simulink library "LopesDevelopmentLibrary"  (R2015b)
settings: Solver=ode45  StartTime=0.0  StopTime=10.0  RelTol=1e-3
values from neighbouring files (symbols this model uses):
  d2r = @(d) d*(pi/180)    [LopesDevelopmentLibrary_LoadParameters.m]
  ts = LopesParams.ts    [LopesDevelopmentLibrary_LoadParameters.m]
undefined symbols (not defined in the file or in its folder): anyParameterChanged, DiscIntNeverNeededParam, gcbh, LAP, LHF, LKF, LopesParams, macaddr, mxpcnetworkconfig, mxpcrtudprx, mxpcrtudptx, patientParametersChanged, port, PX, PZ, RAP, RHF, RKF, SelectorLOPESInSize, StrideTime_s, Time
undefined symbols (not defined in the file): LopesParamsSendDataArrayLen
libraries: LopesDevelopmentLibrary x327, simulink x100, dspmtrx3 x49, xpciplib x6, xpcnetworkbufferlib x5, dspsigops x4, dspstat3 x3, xpcethernetlib x2, visionstatistics x2, xpcseriallib x2, LopesDevelopmentLibraryTest x1, nmc x1
(part 1 of 12)
settings Model: xpc_rtwmakecfg_data=_xpcnblib__xpciplib__xpcetherlib__xpcether8255xlib__xpcetherGbElib_  Creator=Administrator  LastModifiedBy=brugtjh
settings DataIOCC: SaveFormat=Array  SignalLoggingSaveFormat=ModelDataLogs
settings OptimizationCC: ExpressionDepthLimit=2147483647
settings DebuggingCC: UnderspecifiedInitializationDetection=Classic  MergeDetectMultiDrivingBlocksExec=none  SolverPrmCheckMsg=warning  FcnCallInpInsideContextMsg=UseLocalSettings  StateNameClashWarn=warning
settings HardwareCC: ProdBitPerPointer=32  ProdLargestAtomicFloat=None  ProdIntDivRoundTo=Undefined  ProdEndianess=Unspecified  ProdWordSize=32  ProdHWDeviceType=32-bit Generic
settings GRTTargetCC: GeneratePreprocessorConditionals=Disable all  CombineOutputUpdateFcns=off  GRTInterface=on
settings ConfigComp: CovModelRefEnable=Off

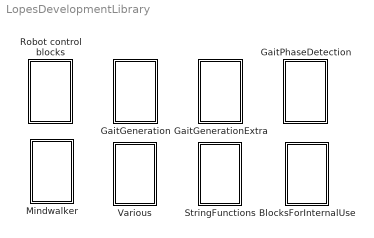
== system LopesDevelopmentLibrary ==
  BlocksForInternalUse : Subsystem
  GaitGeneration : Subsystem
  GaitGenerationExtra : Subsystem
  GaitPhaseDetection : Subsystem
  Mindwalker : Subsystem
  Robot control blocks : Subsystem
  StringFunctions : Subsystem
  Various : Subsystem

== system LopesDevelopmentLibrary/BlocksForInternalUse ==
  GaitGeneration : Subsystem
  GaitGenerationStartStop : Subsystem
  LLC Communication : Subsystem

== system LopesDevelopmentLibrary/GaitGeneration ==
  CalculateBreaksCoefs : Subsystem  TreatAsAtomicUnit=on
  CalculateReferenceStiffnesses : Subsystem
  ConvertStiffness : Subsystem
  GaitParameters : Subsystem
  GeneratePhaseSignalNoFeedback : Subsystem
  GenerateReferenceTrajectory : Subsystem
  PatientParameters : Subsystem
  PhaseEstimatorAoyagi : Subsystem  mask{Weights=[1.0, 0.3, 1.0, 0.3, 0.1, 0, 0.1, 0], AoyagiFilterGain=5}
      mask prompts: Weights "Weights (LHF LKF RHF RKF dLHF dLKF dRHF dRKF) (default: [1.0, 0.3, 1.0, 0.3, 0.1, 0, 0.1, 0])"; AoyagiFilterGain "Aoyagi Filter Gain (default: 5)"
  PhaseEstimatorAoyagi_wPI : Subsystem  mask{Weights=[1.0, 0.1, 1.0, 0.1, 0.0, 0, 0.0, 0], AoyagiFilterGain=2, AoyagiIntegralTimeConstant=5}
      mask prompts: Weights "Weights (LHF LKF RHF RKF dLHF dLKF dRHF dRKF) (default: [1.0, 0.3, 1.0, 0.3, 0.1, 0, 0.1, 0])"; AoyagiFilterGain "Aoyagi Filter Gain (default: 5)"; AoyagiIntegralTimeConstant "Aoyagi Integral Time Constant"

== system LopesDevelopmentLibrary/GaitGenerationExtra ==
  CalculateBreaksCoefs : Subsystem  TreatAsAtomicUnit=on
  GaitGenerationAndAnalysis : Subsystem
      settings: MinAlgLoopOccurrences=on
  GaitParameters : Subsystem
  PhaseEstimatorAoyagi_wPI_Extra : Subsystem  mask{Weights=[1.0, 0.1, 1.0, 0.1, 0.0, 0, 0.0, 0], AoyagiFilterGain=2, AoyagiIntegralTimeConstant=5}
      mask prompts: Weights "Weights (LHF LKF RHF RKF dLHF dLKF dRHF dRKF) (default: [1.0, 0.3, 1.0, 0.3, 0.1, 0, 0.1, 0])"; AoyagiFilterGain "Aoyagi Filter Gain (default: 5)"; AoyagiIntegralTimeConstant "Aoyagi Integral Time Constant"
  VelocityHold : Subsystem

== system LopesDevelopmentLibrary/GaitPhaseDetection ==
  Gait Phase Detection with Wrapper : Subsystem
  Gait Phase detection : Subsystem

== system LopesDevelopmentLibrary/Mindwalker ==
  Mindwalker_AdaptiveTreadmillVelocity : Subsystem
  Mindwalker_Lopes_Conversion : Subsystem

== system LopesDevelopmentLibrary/Robot control blocks ==
  FromLopes : Subsystem
  GeneralLopes : Subsystem  LoadFcn=LopesDevelopmentLibrary_LoadParameters
  RS232SyncBox : Subsystem
  ToLopes : Subsystem

== system LopesDevelopmentLibrary/StringFunctions ==
  Pad : Subsystem  mask{outArrayLen=100}
      mask prompts: outArrayLen "Size of output array"
  PadStrAsDouble : Subsystem  mask{outArrayLen=LopesParams.exceptionStrArrayLen}
      mask prompts: outArrayLen "Size of output array"
  ShowStringInMatlabConsoleIfNotEmpty : MATLAB Function  TreatAsAtomicUnit=on
  concat : MATLAB Function  TreatAsAtomicUnit=on
  concat3 : MATLAB Function  TreatAsAtomicUnit=on
  concat5 : Subsystem  mask{outStrLen=LopesParamsSendDataArrayLen}
      mask prompts: outStrLen "Length of output array"
  concatDelimiter : MATLAB Function  TreatAsAtomicUnit=on
  concatWithOptionalDelimiter : MATLAB Function  TreatAsAtomicUnit=on
  strlen : MATLAB Function  TreatAsAtomicUnit=on
  strlen_as_double : MATLAB Function  TreatAsAtomicUnit=on

== system LopesDevelopmentLibrary/Various ==
  note: Note: I have had problems
      | with real boolean constants
      | in xPC Target. Consider
      | using the Boolean1, which ouptuts
      | a double (and can be converted to boolean
      | if you need to).
  AddToMatrixColumn : Subsystem  mask{col=1, minimum=-inf, maximum=inf}
      mask prompts: col "Column (1-based)"
      mask Display:
      | plot([15,10,10,15],[0,0,75,75])
      | plot([70,75,75,70],[0,0,75,75])
      | plot(0,-5)
      | plot(85,85)
      | plot([55,55],[60,70])
      | plot([50,60],[65,65])
      | plot([55,55],[35,45])
      | plot([50,60],[40,40])
      | plot([55,55],[10,20])
      | plot([50,60],[15,15])
  AddToMatrixElement : Subsystem  mask{row=1, col=1, minimum=-inf, maximum=inf}
      mask prompts: row "Row (1-based)"; col "Column (1-based)"
      mask Display:
      | plot([15,10,10,15],[0,0,75,75])
      | plot([70,75,75,70],[0,0,75,75])
      | plot(0,-5)
      | plot(85,85)
      | plot([55,55],[70,60])
      | plot([50,60],[65,65])
  AdjustAmplitude : Subsystem
  AnyChanged : Subsystem
  AssignMatrixElement : Subsystem  mask{row=3, col=2, minimum=-inf, maximum=inf}
      mask prompts: row "Row (1-based)"; col "Column (1-based)"; minimum "Minimum value"; maximum "Maximum value"
      mask Display:
      | plot([15,10,10,15],[0,0,75,75])
      | plot([70,75,75,70],[0,0,75,75])
      | plot(0,-5)
      | plot(85,85)
      | plot([50,60,60,50,50],[60,60,70,70,60])
  BetterSpringVelocities : Subsystem
  Boolean : Constant  Value=false  OutDataTypeStr=boolean
      settings: OpenFcn=|
      | b = get_param(gcb,'value');
      | if (strcmp(b,'true')),
      |   set_param (gcb,'value','false');
      | else
      |   set_param(gcb,'value','true');
      | end;
  Boolean1 : Constant  Value=0  OutDataTypeStr=double
      settings: OpenFcn=|
      | b = get_param(gcb,'value');
      | if (strcmp(b,'1')),
      |   set_param (gcb,'value','0');
      | else
      |   set_param(gcb,'value','1');
      | end;
  CompareAny : Subsystem  mask{values=[3,4]}
      mask Display: disp(['==(',num2strjoin(values,'||'),')'])
  CrossFade : Subsystem
  CrossfadeInNSeconds : Subsystem
  Cycloid : Subsystem
  Decimation : Subsystem  mask{Decimation=1}
      mask prompts: Decimation "Decimation Amount"
      mask TypeOptions Decimation: DecimationAmount/Value
      mask Display: disp(['Decimation: ',num2str(eval(get_param([gcb,'/DecimationAmount'],'Value')))])
  FilteredDerivative : Subsystem  mask{w=10*(2*pi), z=0.7}
      mask prompts: w "Cut off omega [rad/s]"; z "Zeta"
  FirstOrderLowPassFilter : Subsystem  mask{Tau=1}
  GenerateSyncPulseFromPhase : Subsystem
  IsFirstSample : Subsystem  InitFcn=|
      | return; %Disable this becasue it doesnt work!                                                                                                                                                          
      | h = gcb;                                                                                                                                                                                               
      | n = 0; % Number of enable blocks detected upstream                                                                                                                                                     
      | t = []; % type of enable blocks                                                                                                                                                                        
      | while 1,                                                                                                                                                                                               
      |   % Find parent                                                                                                                                                                                        
      |   h = get_param(h,'parent');                                                                                                                                                                           
      |   if (strcmp(h,'')),                                                                                                                                                                                   
      |       % Then we've reached the root                                                                                                                                                                    
      |       break;                                                                                                                                                                                           
      |   end;                                                                                                                                                                                                 
      |   % and check if it has an enable port                                                                                                                                                                 
      |   e = find_system(h,'searchdepth',1, 'BlockType','EnablePort');                                                                                                                                        
      |   if (numel(e)==1),                                                                                                                                                                                    
      |     s = get_param(e{1},'StatesWhenEnabling');                                                                                                                                                          
      |     n=n+1;                                                                                                                                                                                             
      |     if (strcmp(s,'held')),                                                                                                                                                                             
      |         t=[t;'h']; %#ok<AGROW>                                                                                                                                                                         
      |     else                                                                                                                                                                                               
      |         t=[t;'r']; %#ok<AGROW>                                                                                                                                                                         
      |     end;                                                                                                                                                                                               
      |   elseif (numel(e)>1),                                                                                                                                                                                 
      |       error('hun? Multiple enable blocks!')                                                                                                                                                            
      |   end;                                                                                                                                                                                                 
      | end;                                                                                                                                                                                                   
      |                                                                                                                                                                                                        
      | if (n==0),                                                                                                                                                                                             
      |     warning('Warning: %s - The block is not inside an enabled block',gcb)                                                                                                                              
      | elseif (n==1),                                                                                                                                                                                         
      |     if (t(1)=='r')                                                                                                                                                                                     
      |         % This is okay, do nothing                                                                                                                                                                     
      |     else                                                                                                                                                                                               
      |         warning('Warning: %s - This block is inside an enabled block which has its "State when enabling" set to "held". Usually you want it set to "reset" for correct operation.',gcb);               
      |     end;                                                                                                                                                                                               
      | else % n>1                                                                                                                                                                                             
      |     warning('Warning: %s - This block is inside multiple nested enabled blocks. Check which blocks are "held" and which are "reset". You usually want to have at least one "reset" enabled block',gcb);
      | end;
  Latch : Subsystem  mask{ic=0}
      mask prompts: ic "Initial Condition"
  MonoStable : Constant  Value=0
      settings: OpenFcn=set_param(gcb,'Value','1');tname = ['toggletimer_' gcb];delete(timerfind('name',tname));t = timer('timerfcn', ['set_param(''',gcb,''',''Value'',''0'')'],'executionmode','singleshot','startdelay',3,'name',tname);start(t);
      mask Display: fprintf('PushToTrigger\n%s',get_param(gcb,'value'))
  MultiplyMatrixElement : Subsystem  mask{row=1, col=1, minimum=-inf, maximum=inf}
      mask prompts: row "Row (1-based)"; col "Column (1-based)"; minimum "Minimum value"; maximum "Maximum value"
      mask Display:
      | plot([15,10,10,15],[0,0,75,75])
      | plot([70,75,75,70],[0,0,75,75])
      | plot(0,-5)
      | plot(85,85)
      | plot([50,60],[70,60])
      | plot([50,60],[60,70])
  PhaseShifter1 : Subsystem
  PhaseShifter2 : Subsystem
  PhaseWrapper : Subsystem
  PhaseWrapperAroundZero : Subsystem
  RateLimiterWithBypass : Subsystem  mask{up=3, down=-3}
      mask prompts: up "Rising slew rate:"; down "Falling slew rate:"
      mask help: If Bypass is nonzero, the rate-limiting functionality is bypassed, and the output is made equal to the input immediately.
  RateLimiterWithReset : Subsystem
  RelayCardControl : S-Function  FunctionName=PCI_1761_Relay  Parameters=baseaddress  SFunctionDeploymentMode=off  EnableBusSupport=off  mask{baseaddress=hex2dec('e000')}
      mask prompts: baseaddress "PCI Base Address (e.g. 0x0300)"
  SLRTMessage : Subsystem
  SafeDivide : Subsystem
      mask Display:
      | port_label('input',1,'X')
      | port_label('input',2,'/')
      | port_label('output',1,'')
  Sample Number Generator : Subsystem
      mask Display: disp('Sample Number\nGenerator')
  SampleNoStore : DataStoreMemory  DataStoreName=SAMPLENO  ReadBeforeWriteMsg=warning  WriteAfterWriteMsg=warning  WriteAfterReadMsg=warning
  SampleNumber : Subsystem
  SecondOrderHighPassFilter : Subsystem  mask{w=10*(2*pi), z=0.7}
      mask prompts: w "Cut off omega [rad/s]"; z "Zeta"
  SecondOrderLowPassFilter : Subsystem  mask{w=10*(2*pi), z=0.7}
      mask prompts: w "Cut off omega [rad/s]"; z "Zeta"
  Split : Subsystem
  Stopwatch : Subsystem
  TriggerAtPhaseCrossing : Subsystem
  WeightedAverage : Subsystem

== system LopesDevelopmentLibrary/BlocksForInternalUse/GaitGeneration ==
  CalculateCartesianPositions : Subsystem
  CalculateReferenceGait : Subsystem  TreatAsAtomicUnit=on
  CalculateStiffnessForOneJoint : Subsystem
  OrderKeyEvents : Subsystem
  RegressionData2KeyEvents : Subsystem
  SmoothlyRemove2ndKE : Subsystem
  TrajectoryOfInfluence : Subsystem
  keyEvents2breakscoefs3 : Subsystem  TreatAsAtomicUnit=on
      mask Display:
      | port_label('input',1,'keyEvents')
      | port_label('output',1,'breaks')
      | port_label('output',2,'coefs')
      | disp('keyEvents2breaksCoefs\n3rd order')
  keyEvents2breakscoefs5 : Subsystem  TreatAsAtomicUnit=on
      mask Display:
      | port_label('input',1,'keyEvents')
      | port_label('output',1,'breaks')
      | port_label('output',2,'coefs')
      | disp('keyEvents2breaksCoefs\n5th order')
  ppval_bus : Subsystem  TreatAsAtomicUnit=on

== system LopesDevelopmentLibrary/BlocksForInternalUse/GaitGenerationStartStop ==
  AddUselessKE : Subsystem
  AddUselessKEValue : Subsystem
  CalculateKEforStartup : Subsystem
  "ExtraKeyPoints " : Subsystem  mask{ExtraData='StartLeft', ConnectionPoint=100, SetVelocity=0.3, SetStrideTime=2}
      mask prompts: ExtraData "Name of the extra parameters (IE StartupLeft)"; ConnectionPoint "Connection point:"; SetVelocity "Set Velocity: (0 =  use current velocity)"; SetStrideTime "Set Stride Time: (0 =  use current stride time)"
      mask init:
      | set_param([gcb,'/PelvisTPX/RegressionData'],'Value',['LopesParams.GaitData',ExtraData,'.PX'])
      | set_param([gcb,'/PelvisTPZ/RegressionData'],'Value',['LopesParams.GaitData',ExtraData,'.PZ'])
      | 
      | set_param([gcb,'/LeftHipFlexion/RegressionData'],'Value',['LopesParams.GaitData',ExtraData,'.LHF'])
      | set_param([gcb,'/LeftKneeFlexion/RegressionData'],'Value',['LopesParams.GaitData',ExtraData,'.LKF'])
      | set_param([gcb,'/LeftAnklePF/RegressionData'],'Value',['LopesParams.GaitData',ExtraData,'.LAP'])
      | 
      | set_param([gcb,'/RightHipFlexion/RegressionData'],'Value',['LopesParams.GaitData',ExtraData,'.RHF'])
      | set_param([gcb,'/RightKneeFlexion/RegressionData'],'Value',['LopesParams.GaitData',ExtraData,'.RKF'])
      | set_param([gcb,'/RightAnklePF/RegressionData'],'Value',['LopesParams.GaitData',ExtraData,'.RAP'])
      mask DialogControl DescTextVar Prompt: This Mask sets the Settings for the extra added KeyPoints
  OrderKeyEventsAddOne : Subsystem

== system LopesDevelopmentLibrary/BlocksForInternalUse/LLC Communication ==
  LLC Network Configuration : Subsystem
  LLCReceiveUDP : Subsystem  mask{port=LopesParams.Communication.channel1ReceivePort}
      mask prompts: port "Receive port"
  LLCSendUDP : Subsystem  mask{port=LopesParams.Communication.channel1SendPort}
      mask prompts: port "Send port"
  UDP_Blocks : Subsystem
      mask Display: disp('')

== system LopesDevelopmentLibrary/GaitGeneration/CalculateBreaksCoefs ==
  Parameters : Inport
  Bus Assignment : BusAssignment  AssignedSignals=AnyValueHasChanged
  Bus Selector : BusSelector  OutputSignals=anyParameterChanged
  Calculate : Subsystem
  Data Type Conversion : DataTypeConversion  OutDataTypeStr=double
  BreaksCoefs : Outport  InitialOutput=0
  KeyEventTimes : Outport  Port=2
  Error : Outport  Port=3
  wires:
  Data Type Conversion/1 -> Bus Assignment/2
  Parameters/1 -> Bus Selector/1, Calculate/1(Parameters)
  Calculate/1(BreaksCoefs) -> Bus Assignment/1
  Calculate/2(KeyEventTimes) -> KeyEventTimes/1
  Calculate/3(Error) -> Error/1
  Bus Selector/1 -> Calculate/Enable, Data Type Conversion/1  "<anyParameterChanged>"
  Bus Assignment/1 -> BreaksCoefs/1

== system LopesDevelopmentLibrary/GaitGeneration/CalculateReferenceStiffnesses ==
  note: LHA1 and RHA1 can be used as a starting point
      | for stiffness implementation. They don't work as desired for now,
      | because stiffness for foot placement should increased
      | before heel contact; the key event from LAnkleZ which is used
      | inside the block, is too late.
  Phase : Inport
  KeyEventTimes : Inport  Port=2
  Parameters : Inport  Port=3
  Bus Selector{1,3..15} (14 alike) : BusSelector  OutputSignals=GuidanceForce_pct
  Bus Selector : BusSelector  OutputSignals=RAP,RKF,RHF,LAP,LKF,LHF
  Bus Selector2 : BusSelector  OutputSignals=General,WeightShift,LeftStepHeight,LeftCircumduction,LeftStabilityStance,LeftPrepositioning,LeftSteplength,LeftPushoff,RightStepHeight,RightCircumduction,RightStabilityStance,RightPrepositioning,RightSteplength,RightPushoff
  LAP : Subsystem
  LHA : Subsystem
  LHA1 : Subsystem  Commented=on
  LHF : Subsystem
  LKF : Subsystem
  Mux : Mux  Inputs=10
  PX : Subsystem
  PZ : Subsystem
  RAP : Subsystem
  RHA : Subsystem
  RHA1 : Subsystem  Commented=on
  RHF : Subsystem
  RKF : Subsystem
  Terminator : Terminator
  Terminator1 : Terminator
  Stiffness_pct : Outport
  wires:
  KeyEventTimes/1 -> Bus Selector/1
  Bus Selector15/1 -> Terminator1/1  "<GuidanceForce_pct>"
  Bus Selector14/1 -> Terminator/1  "<GuidanceForce_pct>"
  Bus Selector2/10 -> Bus Selector15/1  "<RightCircumduction>"
  Bus Selector2/4 -> Bus Selector14/1  "<LeftCircumduction>"
  Parameters/1 -> Bus Selector2/1
  Bus Selector4/1 -> PZ/2(WeightShift_GuidanceForce), LHA/1(WeightShift_GuidanceForce), RHA/1(WeightShift_GuidanceForce)  "<GuidanceForce_pct>"
  Bus Selector3/1 -> PZ/1(General_GuidanceForce), LHF/1(General_GuidanceForce), LKF/1(General_GuidanceForce), LAP/1(General_GuidanceForce), RHF/1(General_GuidanceForce), RKF/1(General_GuidanceForce), RAP/1(General_GuidanceForce), PX/1(General_GuidanceForce)  "<GuidanceForce_pct>"
  Mux/1 -> Stiffness_pct/1
  Phase/1 -> RHF/3(phase), RAP/3(phase), RKF/3(phase), LAP/3(phase), LHF/3(phase), LKF/3(phase)
  Bus Selector/5 -> LKF/2(breaks)  "<LKF>"
  Bus Selector/6 -> LHF/2(breaks)  "<LHF>"
  Bus Selector/3 -> RHF/2(breaks)  "<RHF>"
  Bus Selector/2 -> RKF/2(breaks)  "<RKF>"
  LKF/1(Stiffness_pct) -> Mux/5
  LHF/1(Stiffness_pct) -> Mux/4
  RHA/1(Stiffness_pct) -> Mux/7
  LHA/1(Stiffness_pct) -> Mux/3
  RHF/1(Stiffness_pct) -> Mux/8
  PZ/1(Stiffness_pct) -> Mux/2
  RKF/1(Stiffness_pct) -> Mux/9
  PX/1(Stiffness_pct) -> Mux/1
  Bus Selector2/1 -> Bus Selector3/1  "<General>"
  Bus Selector2/2 -> Bus Selector4/1  "<WeightShift>"
  Bus Selector2/3 -> Bus Selector1/1  "<LeftStepHeight>"
  Bus Selector2/6 -> Bus Selector5/1  "<LeftPrepositioning>"
  Bus Selector2/7 -> Bus Selector7/1  "<LeftSteplength>"
  Bus Selector2/9 -> Bus Selector8/1  "<RightStepHeight>"
  Bus Selector2/12 -> Bus Selector9/1  "<RightPrepositioning>"
  Bus Selector2/13 -> Bus Selector11/1  "<RightSteplength>"
  Bus Selector5/1 -> LAP/5(FootPlacement_GuidanceForce), LKF/6(FootPlacement_GuidanceForce), LHF/4(FootPlacement_GuidanceForce)  "<GuidanceForce_pct>"
  Bus Selector7/1 -> LHF/5(StepLength_GuidanceForce)  "<GuidanceForce_pct>"
  Bus Selector1/1 -> LAP/4(StepHeight_GuidanceForce), LKF/4(StepHeight_GuidanceForce)  "<GuidanceForce_pct>"
  Bus Selector13/1 -> LKF/5(StabilityInStance_GuidanceForce)  "<GuidanceForce_pct>"
  Bus Selector2/5 -> Bus Selector13/1  "<LeftStabilityStance>"
  Bus Selector2/11 -> Bus Selector12/1  "<RightStabilityStance>"
  Bus Selector9/1 -> RHF/4(FootPlacement_GuidanceForce), RKF/6(FootPlacement_GuidanceForce), RAP/5(FootPlacement_GuidanceForce)  "<GuidanceForce_pct>"
  Bus Selector11/1 -> RHF/5(StepLength_GuidanceForce)  "<GuidanceForce_pct>"
  Bus Selector8/1 -> RKF/4(StepHeight_GuidanceForce), RAP/4(StepHeight_GuidanceForce)  "<GuidanceForce_pct>"
  Bus Selector12/1 -> RKF/5(StabilityInStance_GuidanceForce)  "<GuidanceForce_pct>"
  RAP/1(Stiffness_pct) -> Mux/10
  LAP/1(Stiffness_pct) -> Mux/6
  Bus Selector/4 -> LAP/2(breaks)  "<LAP>"
  Bus Selector/1 -> RAP/2(breaks)  "<RAP>"
  Bus Selector2/8 -> Bus Selector6/1  "<LeftPushoff>"
  Bus Selector6/1 -> LAP/6(PushOff_GuidanceForce)  "<GuidanceForce_pct>"
  Bus Selector2/14 -> Bus Selector10/1  "<RightPushoff>"
  Bus Selector10/1 -> RAP/6(PushOff_GuidanceForce)  "<GuidanceForce_pct>"

== system LopesDevelopmentLibrary/GaitGeneration/ConvertStiffness ==
  note: This block converts from stiffness-in-percent to stiffness in Nm/rad and N/m.
      | The conversion from Stiffness_pct to Stiffness is nonlinear:
      | S = (S_pct/100)^gamma * MaxStiffness.
  Stiffness_pct : Inport
  ApplyGamma : Math  Operator=pow  SaturateOnIntegerOverflow=on
  Gamma : Constant  Value=LopesParams.Stiffness.Gamma
  MaximumJointStiffness : Constant  Value=LopesParams.Stiffness.MaxJointStiffness
  Product : Product  RndMeth=Zero
  ToFraction : Gain  Gain=0.01
  Stiffness : Outport  LockScale=on
  wires:
  Product/1 -> Stiffness/1
  ApplyGamma/1 -> Product/2
  ToFraction/1 -> ApplyGamma/1
  MaximumJointStiffness/1 -> Product/1
  Gamma/1 -> ApplyGamma/2
  Stiffness_pct/1 -> ToFraction/1

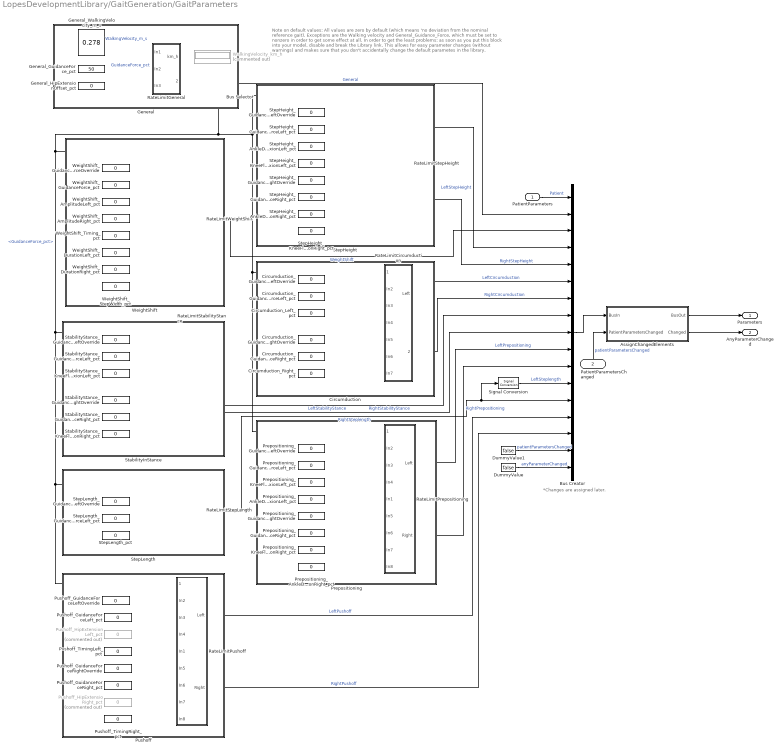
== system LopesDevelopmentLibrary/GaitGeneration/GaitParameters ==
  note: Note on default values:
      | All values are zero by default (which means 'no deviation from the nominal reference gait).
      | Exceptions are the Walking velocity and General_Guidance_Force, which must be
      | set to nonzero in order to get some effect at all.
      |
      | In order to get the least problems: as soon as you put this block into your model, disable and
      | break the Library link. This allows for easy parameter changes (without warnings) and makes
      | sure that you don't accidentally change the default parametes in the library.
  note: *Changes are assigned later.
  PatientParameters : Inport
  PatientParametersChanged : Inport  Port=2
  AssignChangedElements : Subsystem
  Bus Creator : BusCreator  Inputs=17
  Bus Selector : BusSelector  OutputSignals=GuidanceForce_pct
  Circumduction : Subsystem
  Circumduction_GuidanceForceLeftOverride : Constant  Value=0  OutDataTypeStr=double
      settings: OpenFcn=|
      | b = get_param(gcb,'value');
      | if (strcmp(b,'1')),
      |   set_param (gcb,'value','0');
      | else
      |   set_param(gcb,'value','1');
      | end;
  Circumduction_GuidanceForceLeft_pct : Constant  Value=0
  Circumduction_GuidanceForceRightOverride : Constant  Value=0  OutDataTypeStr=double
      settings: OpenFcn=|
      | b = get_param(gcb,'value');
      | if (strcmp(b,'1')),
      |   set_param (gcb,'value','0');
      | else
      |   set_param(gcb,'value','1');
      | end;
  Circumduction_GuidanceForceRight_pct : Constant  Value=0
  Circumduction_Left_pct : Constant  Value=0
  Circumduction_Right_pct : Constant  Value=0
  DummyValue : Constant  Value=false  OutDataTypeStr=boolean
  DummyValue1 : Constant  Value=false
  General : Subsystem
  General_GuidanceForce_pct : Constant  Value=50
  General_HipExtensionOffset_pct : Constant  Value=0
  General_WalkingVelocity_m_s : Constant  Value=0.278
  Prepositioning : Subsystem
  Prepositioning_AnkleDorsiFlexionLeft_pct : Constant  Value=0
  Prepositioning_AnkleDorsiFlexionRight_pct : Constant  Value=0
  Prepositioning_GuidanceForceLeftOverride : Constant  Value=0  OutDataTypeStr=double
      settings: OpenFcn=|
      | b = get_param(gcb,'value');
      | if (strcmp(b,'1')),
      |   set_param (gcb,'value','0');
      | else
      |   set_param(gcb,'value','1');
      | end;
  Prepositioning_GuidanceForceLeft_pct : Constant  Value=0
  Prepositioning_GuidanceForceRightOverride : Constant  Value=0  OutDataTypeStr=double
      settings: OpenFcn=|
      | b = get_param(gcb,'value');
      | if (strcmp(b,'1')),
      |   set_param (gcb,'value','0');
      | else
      |   set_param(gcb,'value','1');
      | end;
  Prepositioning_GuidanceForceRight_pct : Constant  Value=0
  Prepositioning_KneeFlexionLeft_pct : Constant  Value=0
  Prepositioning_KneeFlexionRight_pct : Constant  Value=0
  Pushoff : Subsystem
  Pushoff_GuidanceForceLeftOverride : Constant  Value=0  OutDataTypeStr=double
      settings: OpenFcn=|
      | b = get_param(gcb,'value');
      | if (strcmp(b,'1')),
      |   set_param (gcb,'value','0');
      | else
      |   set_param(gcb,'value','1');
      | end;
  Pushoff_GuidanceForceLeft_pct : Constant  Value=0
  Pushoff_GuidanceForceRightOverride : Constant  Value=0  OutDataTypeStr=double
      settings: OpenFcn=|
      | b = get_param(gcb,'value');
      | if (strcmp(b,'1')),
      |   set_param (gcb,'value','0');
      | else
      |   set_param(gcb,'value','1');
      | end;
  Pushoff_GuidanceForceRight_pct : Constant  Value=0
  Pushoff_HipExtensioRight_pct : Constant  Commented=on  Value=0
  Pushoff_HipExtensionLeft_pct : Constant  Commented=on  Value=0
  Pushoff_TimingLeft_pct : Constant  Value=0
  Pushoff_TimingRight_pct : Constant  Value=0
  RateLimitCircumduction : Subsystem
  RateLimitGeneral : Subsystem
  RateLimitPrepositioning : Subsystem
  RateLimitPushoff : Subsystem
  RateLimitStabilityStance : Subsystem
  RateLimitStepHeight : Subsystem
  RateLimitStepLength : Subsystem
  RateLimitWeightShift : Subsystem
  Signal Conversion : SignalConversion
  StabilityInStance : Subsystem
  StabilityStance_GuidanceForceLeftOverride : Constant  Value=0  OutDataTypeStr=double
      settings: OpenFcn=|
      | b = get_param(gcb,'value');
      | if (strcmp(b,'1')),
      |   set_param (gcb,'value','0');
      | else
      |   set_param(gcb,'value','1');
      | end;
  StabilityStance_GuidanceForceLeft_pct : Constant  Value=0
  StabilityStance_GuidanceForceRightOverride : Constant  Value=0  OutDataTypeStr=double
      settings: OpenFcn=|
      | b = get_param(gcb,'value');
      | if (strcmp(b,'1')),
      |   set_param (gcb,'value','0');
      | else
      |   set_param(gcb,'value','1');
      | end;
  StabilityStance_GuidanceForceRight_pct : Constant  Value=0
  StabilityStance_KneeFlexionLeft_pct : Constant  Value=0
  StabilityStance_KneeFlexionRight_pct : Constant  Value=0
  StepHeight : Subsystem
  StepHeight_AnkleDorsiflexionLeft_pct : Constant  Value=0
  StepHeight_AnkleDorsiflexionRight_pct : Constant  Value=0
  StepHeight_GuidanceForceLeftOverride : Constant  Value=0  OutDataTypeStr=double
      settings: OpenFcn=|
      | b = get_param(gcb,'value');
      | if (strcmp(b,'1')),
      |   set_param (gcb,'value','0');
      | else
      |   set_param(gcb,'value','1');
      | end;
  StepHeight_GuidanceForceLeft_pct : Constant  Value=0
  StepHeight_GuidanceForceRightOverride : Constant  Value=0  OutDataTypeStr=double
      settings: OpenFcn=|
      | b = get_param(gcb,'value');
      | if (strcmp(b,'1')),
      |   set_param (gcb,'value','0');
      | else
      |   set_param(gcb,'value','1');
      | end;
  StepHeight_GuidanceForceRight_pct : Constant  Value=0
  StepHeight_KneeFlexionLeft_pct : Constant  Value=0
  StepHeight_KneeFlexionRight_pct : Constant  Value=0
  StepLength : Subsystem
  StepLength_GuidanceForceLeftOverride : Constant  Value=0  OutDataTypeStr=double
      settings: OpenFcn=|
      | b = get_param(gcb,'value');
      | if (strcmp(b,'1')),
      |   set_param (gcb,'value','0');
      | else
      |   set_param(gcb,'value','1');
      | end;
  StepLength_GuidanceForceLeft_pct : Constant  Value=0
  StepLength_pct : Constant  Value=0
  WalkingVelocity_km_h : Display  Commented=on
  WeightShift : Subsystem
  WeightShift_AmplitudeLeft_pct : Constant  Value=0
  WeightShift_AmplitudeRight_pct : Constant  Value=0
  WeightShift_DurationLeft_pct : Constant  Value=0
  WeightShift_DurationRight_pct : Constant  Value=0
  WeightShift_GuidanceForceOverride : Constant  Value=0  OutDataTypeStr=double
      settings: OpenFcn=|
      | b = get_param(gcb,'value');
      | if (strcmp(b,'1')),
      |   set_param (gcb,'value','0');
      | else
      |   set_param(gcb,'value','1');
      | end;
  WeightShift_GuidanceForce_pct : Constant  Value=0
  WeightShift_StepWidth_pct : Constant  Value=0
  WeightShift_Timing_pct : Constant  Value=0
  Parameters : Outport
  AnyParameterChanged : Outport  Port=2
  wires:
  AssignChangedElements/1(BusOut) -> Parameters/1
  Signal Conversion/1 -> Bus Creator/12  "LeftSteplength"
  DummyValue1/1 -> Bus Creator/16  "patientParametersChanged"
  DummyValue/1 -> Bus Creator/17  "anyParameterChanged"
  RateLimitWeightShift/1(Out1) -> Bus Creator/3  "WeightShift"
  PatientParameters/1 -> Bus Creator/1  "Patient"
  RateLimitStepHeight/1(Left) -> Bus Creator/4  "LeftStepHeight"
  RateLimitStepHeight/2(Right) -> Bus Creator/5  "RightStepHeight"
  RateLimitStabilityStance/1(Left) -> Bus Creator/8  "LeftStabilityStance"
  RateLimitStabilityStance/2(Right) -> Bus Creator/9  "RightStabilityStance"
  RateLimitPrepositioning/1(Left) -> Bus Creator/10  "LeftPrepositioning"
  RateLimitPrepositioning/2(Right) -> Bus Creator/11  "RightPrepositioning"
  RateLimitStepLength/1(StepLength) -> Bus Creator/13, Signal Conversion/1  "RightSteplength"
  RateLimitCircumduction/1(Left) -> Bus Creator/6  "LeftCircumduction"
  RateLimitCircumduction/2(Right) -> Bus Creator/7  "RightCircumduction"
  WeightShift_GuidanceForceOverride/1 -> RateLimitWeightShift/2(In2)
  WeightShift_GuidanceForce_pct/1 -> RateLimitWeightShift/3(In3)
  WeightShift_AmplitudeLeft_pct/1 -> RateLimitWeightShift/4(In4)
  WeightShift_AmplitudeRight_pct/1 -> RateLimitWeightShift/5(In5)
  WeightShift_Timing_pct/1 -> RateLimitWeightShift/6(In6)
  WeightShift_DurationLeft_pct/1 -> RateLimitWeightShift/7(In7)
  WeightShift_DurationRight_pct/1 -> RateLimitWeightShift/8(In8)
  WeightShift_StepWidth_pct/1 -> RateLimitWeightShift/9(In9)
  StepHeight_GuidanceForceLeftOverride/1 -> RateLimitStepHeight/2(In2)
  StepHeight_GuidanceForceLeft_pct/1 -> RateLimitStepHeight/3(In3)
  StepHeight_KneeFlexionLeft_pct/1 -> RateLimitStepHeight/5(In4)
  StepHeight_GuidanceForceRightOverride/1 -> RateLimitStepHeight/6(In5)
  StepHeight_GuidanceForceRight_pct/1 -> RateLimitStepHeight/7(In6)
  StepHeight_KneeFlexionRight_pct/1 -> RateLimitStepHeight/9(In7)
  Circumduction_GuidanceForceLeftOverride/1 -> RateLimitCircumduction/2(In2)
  Circumduction_GuidanceForceLeft_pct/1 -> RateLimitCircumduction/3(In3)
  Circumduction_Left_pct/1 -> RateLimitCircumduction/4(In4)
  Circumduction_GuidanceForceRightOverride/1 -> RateLimitCircumduction/5(In5)
  Circumduction_GuidanceForceRight_pct/1 -> RateLimitCircumduction/6(In6)
  Circumduction_Right_pct/1 -> RateLimitCircumduction/7(In7)
  StabilityStance_GuidanceForceLeftOverride/1 -> RateLimitStabilityStance/2(In2)
  StabilityStance_GuidanceForceLeft_pct/1 -> RateLimitStabilityStance/3(In3)
  StabilityStance_KneeFlexionLeft_pct/1 -> RateLimitStabilityStance/4(In4)
  StabilityStance_GuidanceForceRightOverride/1 -> RateLimitStabilityStance/5(In5)
  StabilityStance_GuidanceForceRight_pct/1 -> RateLimitStabilityStance/6(In6)
  StabilityStance_KneeFlexionRight_pct/1 -> RateLimitStabilityStance/7(In7)
  Prepositioning_GuidanceForceLeftOverride/1 -> RateLimitPrepositioning/2(In2)
  Prepositioning_GuidanceForceLeft_pct/1 -> RateLimitPrepositioning/3(In3)
  Prepositioning_KneeFlexionLeft_pct/1 -> RateLimitPrepositioning/4(In4)
  Prepositioning_GuidanceForceRightOverride/1 -> RateLimitPrepositioning/6(In5)
  Prepositioning_GuidanceForceRight_pct/1 -> RateLimitPrepositioning/7(In6)
  Prepositioning_KneeFlexionRight_pct/1 -> RateLimitPrepositioning/8(In7)
  StepLength_GuidanceForceLeftOverride/1 -> RateLimitStepLength/2(In2)
  StepLength_GuidanceForceLeft_pct/1 -> RateLimitStepLength/3(In3)
  StepLength_pct/1 -> RateLimitStepLength/4(In4)
  Bus Selector/1 -> RateLimitStepHeight/1(GeneralGF), RateLimitPrepositioning/1(GeneralGF), RateLimitCircumduction/1(GeneralGF), RateLimitWeightShift/1(GeneralGF), RateLimitPushoff/1(GeneralGF), RateLimitStepLength/1(GeneralGF), RateLimitStabilityStance/1(GeneralGF)  "<GuidanceForce_pct>"
  RateLimitGeneral/2(General) -> Bus Creator/2, Bus Selector/1  "General"
  General_WalkingVelocity_m_s/1 -> RateLimitGeneral/1(In1)  "WalkingVelocity_m_s"
  General_GuidanceForce_pct/1 -> RateLimitGeneral/2(In2)  "GuidanceForce_pct"
  General_HipExtensionOffset_pct/1 -> RateLimitGeneral/3(In3)
  RateLimitGeneral/1(km_h) -> WalkingVelocity_km_h/1
  Bus Creator/1 -> AssignChangedElements/1(BusIn)
  PatientParametersChanged/1 -> AssignChangedElements/2(PatientParametersChanged)  "patientParametersChanged"
  AssignChangedElements/2(Changed) -> AnyParameterChanged/1
  StepHeight_AnkleDorsiflexionLeft_pct/1 -> RateLimitStepHeight/4(In1)
  StepHeight_AnkleDorsiflexionRight_pct/1 -> RateLimitStepHeight/8(In8)
  Prepositioning_AnkleDorsiFlexionLeft_pct/1 -> RateLimitPrepositioning/5(In1)
  Prepositioning_AnkleDorsiFlexionRight_pct/1 -> RateLimitPrepositioning/9(In8)
  Pushoff_GuidanceForceLeft_pct/1 -> RateLimitPushoff/3(In3)
  Pushoff_HipExtensionLeft_pct/1 -> RateLimitPushoff/4(In4)
  Pushoff_GuidanceForceRightOverride/1 -> RateLimitPushoff/6(In5)
  Pushoff_GuidanceForceRight_pct/1 -> RateLimitPushoff/7(In6)
  Pushoff_HipExtensioRight_pct/1 -> RateLimitPushoff/8(In7)
  Pushoff_TimingLeft_pct/1 -> RateLimitPushoff/5(In1)
  Pushoff_TimingRight_pct/1 -> RateLimitPushoff/9(In8)
  RateLimitPushoff/1(Left) -> Bus Creator/14  "LeftPushoff"
  RateLimitPushoff/2(Right) -> Bus Creator/15  "RightPushoff"
  Pushoff_GuidanceForceLeftOverride/1 -> RateLimitPushoff/2(In2)

== system LopesDevelopmentLibrary/GaitGeneration/GeneratePhaseSignalNoFeedback ==
  note: This block is a very simple implementation
      | of a phase-signal generator. You can use this for testing.
      | However, don't use it for real experiments.
      |
      | It seems logical to fix the step time. However, the step length
      | and walking velocity are also fixed. The step time can be uniquely
      | determined from this. If we would also fix the step time, we'd get
      | an overdetermined system. In order to avoid, we need to
      | leave the step time free to change. Therefore, this block
      | (which fixes step time because it fixes phase evolution), should
      | not be used in reality.
  BreaksCoefs : Inport
  Bus Selector2 : BusSelector  OutputSignals=StrideTime_s
  Constant3 : Constant  Value=100
  Integrator : Integrator
  PhaseWrapper : LopesDevelopmentLibrary/Various/PhaseWrapper
  SafeDivide : LopesDevelopmentLibrary/Various/SafeDivide  SystemSampleTime=-1
  Phase_pct : Outport
  PhaseRate_pct_s : Outport  Port=2
  wires:
  BreaksCoefs/1 -> Bus Selector2/1
  Constant3/1 -> SafeDivide/1
  SafeDivide/1 -> Integrator/1, PhaseRate_pct_s/1
  Bus Selector2/1 -> SafeDivide/2  "<StrideTime_s>"
  Integrator/1 -> PhaseWrapper/1
  PhaseWrapper/1 -> Phase_pct/1

== system LopesDevelopmentLibrary/GaitGeneration/GenerateReferenceTrajectory ==
  Phase : Inport
  BreaksCoefs : Inport  Port=2
  Parameters : Inport  Port=3
  Bus Selector : BusSelector  OutputSignals=General.WalkingVelocity_m_s
  CalculateReferenceGait : LopesDevelopmentLibrary/BlocksForInternalUse/GaitGeneration/CalculateReferenceGait
  CopySignal : SignalConversion
  Terminator1 : Terminator
  Terminator2 : Terminator
  JointAngles : Outport
  JointAngularVelocities : Outport  Port=2
  JointAngularAccelerations : Outport  Port=3
  TreadmillVelocity : Outport  Port=4
  TimeSinceLeftHeelstrike : Outport  Port=5
  wires:
  CalculateReferenceGait/6 -> Terminator2/1
  CalculateReferenceGait/5 -> Terminator1/1
  CalculateReferenceGait/1 -> JointAngles/1
  Parameters/1 -> CalculateReferenceGait/3, Bus Selector/1
  BreaksCoefs/1 -> CalculateReferenceGait/2
  CopySignal/1 -> TreadmillVelocity/1
  Phase/1 -> CalculateReferenceGait/1
  CalculateReferenceGait/2 -> JointAngularVelocities/1
  CalculateReferenceGait/3 -> JointAngularAccelerations/1
  CalculateReferenceGait/4 -> TimeSinceLeftHeelstrike/1
  Bus Selector/1 -> CopySignal/1  "<WalkingVelocity_m_s>"

== system LopesDevelopmentLibrary/GaitGeneration/PatientParameters ==
  note: Warning: Only change these values while in state Off.
      | Otherwise, the result may be unexpected (things don't go
      | really wrong, but the results may be less accurate).
  note: Distance between hip joints
  note: Don't change (the ankle of Lopes is 0.1 m above the
      | ground, regardless of where the human's ankle is).
  note: this should be a little shorter than the
      | real foot length. 0.2 to 0.25 is usually best.
  AnyChanged : LopesDevelopmentLibrary/Various/AnyChanged
  BodyLength_m : Constant  Value=1.80
  Bus Creator : BusCreator  Inputs=8
  FootHeight_m : Constant  Value=0.10
  FootLength_m : Constant  Value=0.2
  LowerLegLength_m : Constant  Value=0.5
  Mass_kg : Constant  Value=80
  PelvisHeight_m : Constant  Value=0.2
  PelvisWidth_m : Constant  Value=0.2
  UpperLegLength_m : Constant  Value=0.5
  PatientParameters : Outport
  PatientParametersChanged : Outport  Port=2
  wires:
  PelvisHeight_m/1 -> Bus Creator/8  "PelvisHeight_m"
  PelvisWidth_m/1 -> Bus Creator/7  "PelvisWidth_m"
  FootHeight_m/1 -> Bus Creator/6  "FootHeight_m"
  BodyLength_m/1 -> Bus Creator/1  "BodyLength_m"
  Mass_kg/1 -> Bus Creator/5  "Mass_kg"
  Bus Creator/1 -> AnyChanged/1, PatientParameters/1
  UpperLegLength_m/1 -> Bus Creator/2  "UpperLegLength_m"
  LowerLegLength_m/1 -> Bus Creator/3  "LowerLegLength_m"
  FootLength_m/1 -> Bus Creator/4  "FootLength_m"
  AnyChanged/1 -> PatientParametersChanged/1

== system LopesDevelopmentLibrary/GaitGeneration/PhaseEstimatorAoyagi ==
  note: This block is a phase estimator based on the paper by Aoyagi 2007. It consists of two parts:
      | -  a raw estimator which estimates the current phase simply based on the euclidean distance
      |    to each point on the trajectory (it returns the phase at which this distance is minimum), and
      | - a (sort-of-low-pass)-filter which generates a continuous and not-too-fast-changing output phase.
  MeasuredJointAngles : Inport
  MeasuredJointVelocities : Inport  Port=2
  BreaksCoefs : Inport  Port=3
  ResetHighActive : Inport  Port=4
  Bus Selector : BusSelector  OutputSignals=StrideTime_s
  EstimatePhaseDirectlyAoyagi : Subsystem
  PhaseFilterAoyagi : Subsystem
  EstmiatedPhase_pct : Outport
  EstmiatedPhaseRate_pct_s : Outport  Port=2
  wires:
  MeasuredJointAngles/1 -> EstimatePhaseDirectlyAoyagi/1(MeasuredJointAngles)
  BreaksCoefs/1 -> Bus Selector/1, EstimatePhaseDirectlyAoyagi/3(BreaksCoefs)
  MeasuredJointVelocities/1 -> EstimatePhaseDirectlyAoyagi/2(MeasuredJointVelocities)
  EstimatePhaseDirectlyAoyagi/1(EstimtatedPhaseUnfiltered) -> PhaseFilterAoyagi/1(EstimatedPhaseUnfiltered)
  Bus Selector/1 -> PhaseFilterAoyagi/2(ReferenceStrideTime)  "<StrideTime_s>"
  PhaseFilterAoyagi/1(EstimatedPhase) -> EstmiatedPhase_pct/1
  ResetHighActive/1 -> PhaseFilterAoyagi/3(ResetHighActive)
  PhaseFilterAoyagi/2(EstimatedPhaseRate) -> EstmiatedPhaseRate_pct_s/1

== system LopesDevelopmentLibrary/GaitGeneration/PhaseEstimatorAoyagi_wPI ==
  note: This block is a phase estimator based on the paper by Aoyagi 2007. It consists of two parts:
      | -  a raw estimator which estimates the current phase simply based on the euclidean distance
      |    to each point on the trajectory (it returns the phase at which this distance is minimum), and
      | - a (sort-of-low-pass)-filter which generates a continuous and not-too-fast-changing output phase.
  MeasuredJointAngles : Inport
  MeasuredJointVelocities : Inport  Port=2
  BreaksCoefs : Inport  Port=3
  ResetHighActive : Inport  Port=4
  Bus Selector : BusSelector  OutputSignals=StrideTime_s
  EstimatePhaseDirectlyAoyagi : Subsystem
  PhaseFilterAoyagi : Subsystem
  EstmiatedPhase_pct : Outport
  EstmiatedPhaseRate_pct_s : Outport  Port=2
  wires:
  PhaseFilterAoyagi/2(EstimatedPhaseRate) -> EstmiatedPhaseRate_pct_s/1
  ResetHighActive/1 -> PhaseFilterAoyagi/3(ResetHighActive)
  PhaseFilterAoyagi/1(EstimatedPhase) -> EstmiatedPhase_pct/1
  Bus Selector/1 -> PhaseFilterAoyagi/2(ReferenceStrideTime)  "<StrideTime_s>"
  EstimatePhaseDirectlyAoyagi/1(EstimtatedPhaseUnfiltered) -> PhaseFilterAoyagi/1(EstimatedPhaseUnfiltered)
  MeasuredJointVelocities/1 -> EstimatePhaseDirectlyAoyagi/2(MeasuredJointVelocities)
  BreaksCoefs/1 -> EstimatePhaseDirectlyAoyagi/3(BreaksCoefs), Bus Selector/1
  MeasuredJointAngles/1 -> EstimatePhaseDirectlyAoyagi/1(MeasuredJointAngles)

== system LopesDevelopmentLibrary/GaitGenerationExtra/CalculateBreaksCoefs ==
  Parameters : Inport
  SetState : Inport  Port=2
  Bus Assignment : BusAssignment  AssignedSignals=AnyValueHasChanged
  Bus Selector : BusSelector  OutputSignals=anyParameterChanged
  Calculate : Subsystem
  Data Type Conversion : DataTypeConversion  OutDataTypeStr=double
  Detect Change : simulink/Logic and Bit Operations/Detect Change  vinit=1  InputProcessing=Inherited  OutDataTypeStr=boolean
  Logical Operator : Logic  Operator=OR  AllPortsSameDT=off  OutDataTypeStr=boolean
  BreaksCoefs : Outport  InitialOutput=0
  KeyEventTimes : Outport  Port=2
  Error : Outport  Port=3
  wires:
  Data Type Conversion/1 -> Bus Assignment/2
  Parameters/1 -> Bus Selector/1, Calculate/1(Parameters)
  Calculate/1(BreaksCoefs) -> Bus Assignment/1
  Calculate/2(KeyEventTimes) -> KeyEventTimes/1
  Calculate/3(Error) -> Error/1
  Bus Assignment/1 -> BreaksCoefs/1
  SetState/1 -> Detect Change/1, Calculate/2(State)
  Detect Change/1 -> Logical Operator/2
  Bus Selector/1 -> Logical Operator/1  "<anyParameterChanged>"
  Logical Operator/1 -> Calculate/Enable, Data Type Conversion/1
